simulink model "OpenLoop"  (R2025b)
settings: Solver=VariableStepAuto  StartTime=0.0  StopTime=500  RelTol=1e-3
settings Model: Creator=denni  LastModifiedBy=hakee
settings RTWCC: GPUComputeCapability=3.5

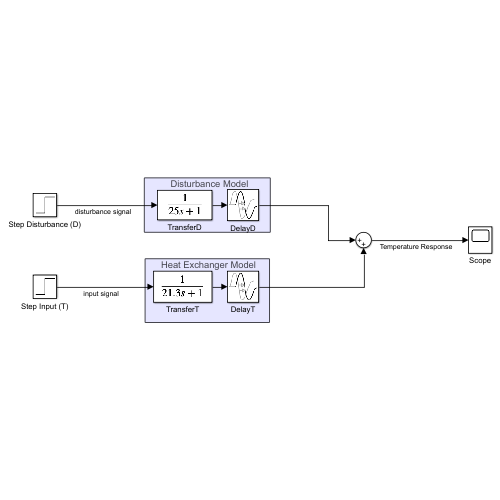
[thumbnail: Simulink's stored preview of the top-level diagram]
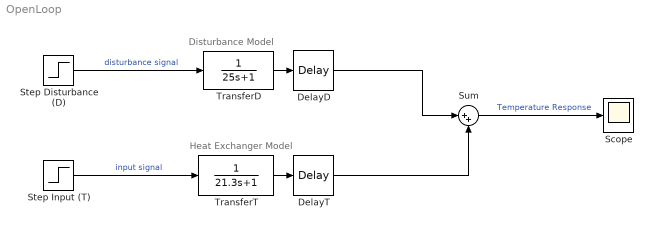
== system OpenLoop ==
  note: Disturbance Model
  note: Heat Exchanger Model
  DelayD : TransportDelay  DelayTime=35
  DelayT : TransportDelay  DelayTime=14.7
  Scope : Scope
      settings: ActiveDisplayYMinimum=-0.5344524255788472  ActiveDisplayYMaximum=2.4388712300300672
  Step Disturbance (D) : Step  Time=0  SampleTime=0
  Step Input (T) : Step  Time=0  SampleTime=0
  Sum : Sum  Inputs=|++
  TransferD : TransferFcn  Denominator=[25 1]  ContinuousStateAttributes='disturbance'
  TransferT : TransferFcn  Denominator=[21.3 1]  ContinuousStateAttributes='heat'
  wires:
  TransferT/1 -> DelayT/1
  TransferD/1 -> DelayD/1
  DelayT/1 -> Sum/2
  Step Disturbance (D)/1 -> TransferD/1  "disturbance signal"
  Step Input (T)/1 -> TransferT/1  "input signal"
  DelayD/1 -> Sum/1
  Sum/1 -> Scope/1  "Temperature Response"
